simulink model "coba1 - Copy"  (R2021a)
settings: Solver=VariableStepAuto  StartTime=0.0  StopTime=200  RelTol=1e-3
undefined symbols (not defined in the file): Ion, Lithium
libraries: spsSeriesRLCBranchLib x23, spsIdealSwitchLib x14, spsBatteryLib x12, spsDiodeLib x12, spsDCVoltageSourceLib x1, spsGroundLib x1, spsPWMGenerator2LevelLib x1, spspowerguiLib x1
settings Model: Creator=jafar  LastModifiedBy=jafar

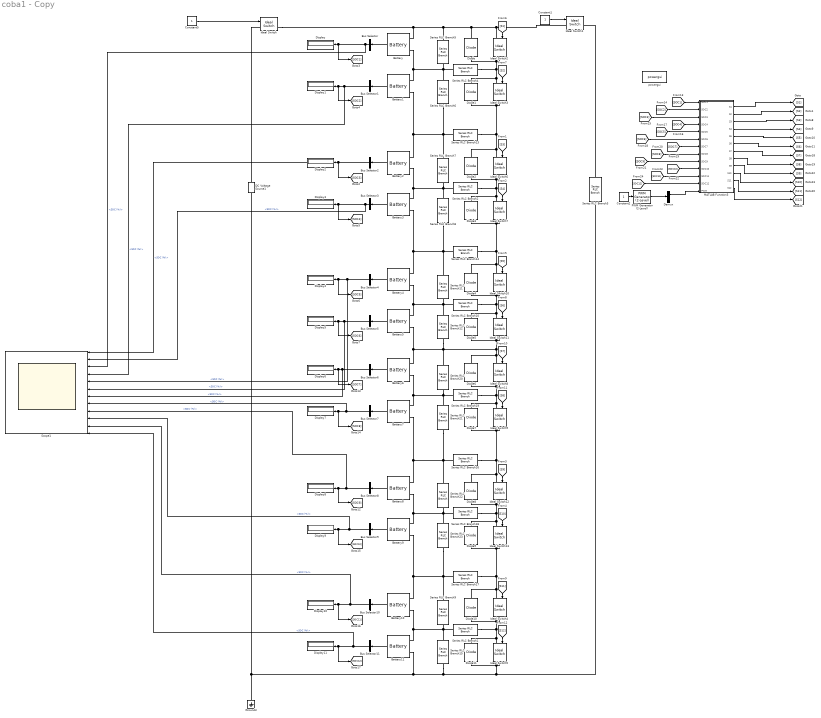
== system coba1 - Copy ==
  Battery : spsBatteryLib/Battery  BatType=Lithium-Ion  ShowTempParam=off  ThermalPreset=no  ShowAgeParam=off  NomV=3.7  NomQ=5.4  SOC=20  Batt_Tr=30  PresetModel=on  MaxQ=5.4  MinV=2.775  FullV=4.3068  Dis_rate=2.3478  R=0.0068519  Normal_OP=4.8835  expZone="[3.9974      0.2653]"  current=[6.5 13 32.5]  Units=Time  Tci=20  NomT=20  T2=-30  MaxQ2=4.8  FullV2=7.1  Normal_OP2=5.655  expZone2="[6.58           1]"  Rca=0.6  ti=2000  Dp=0  Neq0=0  Tsim=1e6  Ta1=25  Qeol=5.4*0.9  Reol=0.013333*1.2  Char_age=[2.3478, 3]  Dis_age=[2.3478, 10]  N1=1500  N2=10500  N3=1000  N4=1400  Ta2=45  N5=950
  Battery1 : spsBatteryLib/Battery  BatType=Lithium-Ion  ShowTempParam=off  ThermalPreset=no  ShowAgeParam=off  NomV=3.7  NomQ=5.4  SOC=30  Batt_Tr=30  PresetModel=on  MaxQ=5.4  MinV=2.775  FullV=4.3068  Dis_rate=2.3478  R=0.0068519  Normal_OP=4.8835  expZone="[3.9974      0.2653]"  current=[6.5 13 32.5]  Units=Time  Tci=20  NomT=20  T2=-30  MaxQ2=4.8  FullV2=7.1  Normal_OP2=5.655  expZone2="[6.58           1]"  Rca=0.6  ti=2000  Dp=0  Neq0=0  Tsim=1e6  Ta1=25  Qeol=5.4*0.9  Reol=0.013333*1.2  Char_age=[2.3478, 3]  Dis_age=[2.3478, 10]  N1=1500  N2=10500  N3=1000  N4=1400  Ta2=45  N5=950
  Battery10 : spsBatteryLib/Battery  BatType=Lithium-Ion  ShowTempParam=off  ThermalPreset=no  ShowAgeParam=off  NomV=3.7  NomQ=5.4  SOC=10  Batt_Tr=30  PresetModel=on  MaxQ=5.4  MinV=2.775  FullV=4.3068  Dis_rate=2.3478  R=0.0068519  Normal_OP=4.8835  expZone="[3.9974      0.2653]"  current=[6.5 13 32.5]  Units=Time  Tci=20  NomT=20  T2=-30  MaxQ2=4.8  FullV2=7.1  Normal_OP2=5.655  expZone2="[6.58           1]"  Rca=0.6  ti=2000  Dp=0  Neq0=0  Tsim=1e6  Ta1=25  Qeol=5.4*0.9  Reol=0.013333*1.2  Char_age=[2.3478, 3]  Dis_age=[2.3478, 10]  N1=1500  N2=10500  N3=1000  N4=1400  Ta2=45  N5=950
  Battery11 : spsBatteryLib/Battery  BatType=Lithium-Ion  ShowTempParam=off  ThermalPreset=no  ShowAgeParam=off  NomV=3.7  NomQ=5.4  SOC=0  Batt_Tr=30  PresetModel=on  MaxQ=5.4  MinV=2.775  FullV=4.3068  Dis_rate=2.3478  R=0.0068519  Normal_OP=4.8835  expZone="[3.9974      0.2653]"  current=[6.5 13 32.5]  Units=Time  Tci=20  NomT=20  T2=-30  MaxQ2=4.8  FullV2=7.1  Normal_OP2=5.655  expZone2="[6.58           1]"  Rca=0.6  ti=2000  Dp=0  Neq0=0  Tsim=1e6  Ta1=25  Qeol=5.4*0.9  Reol=0.013333*1.2  Char_age=[2.3478, 3]  Dis_age=[2.3478, 10]  N1=1500  N2=10500  N3=1000  N4=1400  Ta2=45  N5=950
  Battery2 : spsBatteryLib/Battery  BatType=Lithium-Ion  ShowTempParam=off  ThermalPreset=no  ShowAgeParam=off  NomV=3.7  NomQ=5.4  SOC=40  Batt_Tr=30  PresetModel=on  MaxQ=5.4  MinV=2.775  FullV=4.3068  Dis_rate=2.3478  R=0.0068519  Normal_OP=4.8835  expZone="[3.9974      0.2653]"  current=[6.5 13 32.5]  Units=Time  Tci=20  NomT=20  T2=-30  MaxQ2=4.8  FullV2=7.1  Normal_OP2=5.655  expZone2="[6.58           1]"  Rca=0.6  ti=2000  Dp=0  Neq0=0  Tsim=1e6  Ta1=25  Qeol=5.4*0.9  Reol=0.013333*1.2  Char_age=[2.3478, 3]  Dis_age=[2.3478, 10]  N1=1500  N2=10500  N3=1000  N4=1400  Ta2=45  N5=950
  Battery3 : spsBatteryLib/Battery  BatType=Lithium-Ion  ShowTempParam=off  ThermalPreset=no  ShowAgeParam=off  NomV=3.7  NomQ=5.4  SOC=50  Batt_Tr=30  PresetModel=on  MaxQ=5.4  MinV=2.775  FullV=4.3068  Dis_rate=2.3478  R=0.0068519  Normal_OP=4.8835  expZone="[3.9974      0.2653]"  current=[6.5 13 32.5]  Units=Time  Tci=20  NomT=20  T2=-30  MaxQ2=4.8  FullV2=7.1  Normal_OP2=5.655  expZone2="[6.58           1]"  Rca=0.6  ti=2000  Dp=0  Neq0=0  Tsim=1e6  Ta1=25  Qeol=5.4*0.9  Reol=0.013333*1.2  Char_age=[2.3478, 3]  Dis_age=[2.3478, 10]  N1=1500  N2=10500  N3=1000  N4=1400  Ta2=45  N5=950
  Battery4 : spsBatteryLib/Battery  BatType=Lithium-Ion  ShowTempParam=off  ThermalPreset=no  ShowAgeParam=off  NomV=3.7  NomQ=5.4  SOC=60  Batt_Tr=30  PresetModel=on  MaxQ=5.4  MinV=2.775  FullV=4.3068  Dis_rate=2.3478  R=0.0068519  Normal_OP=4.8835  expZone="[3.9974      0.2653]"  current=[6.5 13 32.5]  Units=Time  Tci=20  NomT=20  T2=-30  MaxQ2=4.8  FullV2=7.1  Normal_OP2=5.655  expZone2="[6.58           1]"  Rca=0.6  ti=2000  Dp=0  Neq0=0  Tsim=1e6  Ta1=25  Qeol=5.4*0.9  Reol=0.013333*1.2  Char_age=[2.3478, 3]  Dis_age=[2.3478, 10]  N1=1500  N2=10500  N3=1000  N4=1400  Ta2=45  N5=950
  Battery5 : spsBatteryLib/Battery  BatType=Lithium-Ion  ShowTempParam=off  ThermalPreset=no  ShowAgeParam=off  NomV=3.7  NomQ=5.4  SOC=70  Batt_Tr=30  PresetModel=on  MaxQ=5.4  MinV=2.775  FullV=4.3068  Dis_rate=2.3478  R=0.0068519  Normal_OP=4.8835  expZone="[3.9974      0.2653]"  current=[6.5 13 32.5]  Units=Time  Tci=20  NomT=20  T2=-30  MaxQ2=4.8  FullV2=7.1  Normal_OP2=5.655  expZone2="[6.58           1]"  Rca=0.6  ti=2000  Dp=0  Neq0=0  Tsim=1e6  Ta1=25  Qeol=5.4*0.9  Reol=0.013333*1.2  Char_age=[2.3478, 3]  Dis_age=[2.3478, 10]  N1=1500  N2=10500  N3=1000  N4=1400  Ta2=45  N5=950
  Battery6 : spsBatteryLib/Battery  BatType=Lithium-Ion  ShowTempParam=off  ThermalPreset=no  ShowAgeParam=off  NomV=3.7  NomQ=5.4  SOC=35  Batt_Tr=30  PresetModel=on  MaxQ=5.4  MinV=2.775  FullV=4.3068  Dis_rate=2.3478  R=0.0068519  Normal_OP=4.8835  expZone="[3.9974      0.2653]"  current=[6.5 13 32.5]  Units=Time  Tci=20  NomT=20  T2=-30  MaxQ2=4.8  FullV2=7.1  Normal_OP2=5.655  expZone2="[6.58           1]"  Rca=0.6  ti=2000  Dp=0  Neq0=0  Tsim=1e6  Ta1=25  Qeol=5.4*0.9  Reol=0.013333*1.2  Char_age=[2.3478, 3]  Dis_age=[2.3478, 10]  N1=1500  N2=10500  N3=1000  N4=1400  Ta2=45  N5=950
  Battery7 : spsBatteryLib/Battery  BatType=Lithium-Ion  ShowTempParam=off  ThermalPreset=no  ShowAgeParam=off  NomV=3.7  NomQ=5.4  SOC=45  Batt_Tr=30  PresetModel=on  MaxQ=5.4  MinV=2.775  FullV=4.3068  Dis_rate=2.3478  R=0.0068519  Normal_OP=4.8835  expZone="[3.9974      0.2653]"  current=[6.5 13 32.5]  Units=Time  Tci=20  NomT=20  T2=-30  MaxQ2=4.8  FullV2=7.1  Normal_OP2=5.655  expZone2="[6.58           1]"  Rca=0.6  ti=2000  Dp=0  Neq0=0  Tsim=1e6  Ta1=25  Qeol=5.4*0.9  Reol=0.013333*1.2  Char_age=[2.3478, 3]  Dis_age=[2.3478, 10]  N1=1500  N2=10500  N3=1000  N4=1400  Ta2=45  N5=950
  Battery8 : spsBatteryLib/Battery  BatType=Lithium-Ion  ShowTempParam=off  ThermalPreset=no  ShowAgeParam=off  NomV=3.7  NomQ=5.4  SOC=30  Batt_Tr=30  PresetModel=on  MaxQ=5.4  MinV=2.775  FullV=4.3068  Dis_rate=2.3478  R=0.0068519  Normal_OP=4.8835  expZone="[3.9974      0.2653]"  current=[6.5 13 32.5]  Units=Time  Tci=20  NomT=20  T2=-30  MaxQ2=4.8  FullV2=7.1  Normal_OP2=5.655  expZone2="[6.58           1]"  Rca=0.6  ti=2000  Dp=0  Neq0=0  Tsim=1e6  Ta1=25  Qeol=5.4*0.9  Reol=0.013333*1.2  Char_age=[2.3478, 3]  Dis_age=[2.3478, 10]  N1=1500  N2=10500  N3=1000  N4=1400  Ta2=45  N5=950
  Battery9 : spsBatteryLib/Battery  BatType=Lithium-Ion  ShowTempParam=off  ThermalPreset=no  ShowAgeParam=off  NomV=3.7  NomQ=5.4  SOC=20  Batt_Tr=30  PresetModel=on  MaxQ=5.4  MinV=2.775  FullV=4.3068  Dis_rate=2.3478  R=0.0068519  Normal_OP=4.8835  expZone="[3.9974      0.2653]"  current=[6.5 13 32.5]  Units=Time  Tci=20  NomT=20  T2=-30  MaxQ2=4.8  FullV2=7.1  Normal_OP2=5.655  expZone2="[6.58           1]"  Rca=0.6  ti=2000  Dp=0  Neq0=0  Tsim=1e6  Ta1=25  Qeol=5.4*0.9  Reol=0.013333*1.2  Char_age=[2.3478, 3]  Dis_age=[2.3478, 10]  N1=1500  N2=10500  N3=1000  N4=1400  Ta2=45  N5=950
  Bus Selector{,1..11} (12 alike) : BusSelector  OutputSignals=SOC (%)
  Constant1 : Constant
  Constant2 : Constant
  Constant5 : Constant
  DC Voltage Source1 : spsDCVoltageSourceLib/DC Voltage Source  Amplitude=72  Measurements=None
  Demux : Demux  Outputs=2
  Diode{,1..11} (12 alike) : spsDiodeLib/Diode  Ron=0.001  Lon=0  Vf=0.8  IC=0  UseSnubber=0  Rs=500  Cs=250e-9  Measurements=off
  Display{,1..11} (12 alike) : Display
  Ground3 : spsGroundLib/Ground  LConnTagsString=a
  Ideal Switch : spsIdealSwitchLib/Ideal Switch  Ron=0.001  Lon=0  IC=0  Rs=1e5  Cs=inf  Measurements=on
  Ideal Switch1 : spsIdealSwitchLib/Ideal Switch  Ron=0.001  Lon=0  IC=0  Rs=1e5  Cs=inf  Measurements=on
  Ideal Switch{2..13} (12 alike) : spsIdealSwitchLib/Ideal Switch  Ron=0.001  Lon=0  IC=0  Rs=1e5  Cs=inf  Measurements=off
  MATLAB Function3 : MATLAB Function  TreatAsAtomicUnit=on
  PWM Generator (2-Level) : spsPWMGenerator2LevelLib/PWM Generator (2-Level)  ModulatorType=Single-phase half-bridge (2 pulses)  ModulatorMode=Unsynchronized  Fc=500  Pc=0  nF=27  MinMax="[ -1  1 ]"  SamplingTechnique=Natural  ModulatingSignals=off  m=0.8  Freq=60  Phase=0  Ts=0  ShowCarrierOutport=off
  Scope1 : Scope  NumInputPorts=12
  Series RLC Branch{1..2,4,10,13..14,16..19} (10 alike) : spsSeriesRLCBranchLib/Series RLC Branch  LConnTagsString=__new0  RConnTagsString=__new0  BranchType=L  Resistance=1  Inductance=1e-3  SetiL0=off  InitialCurrent=0  Capacitance=1e-6  Setx0=off  InitialVoltage=0  Measurements=None
  Series RLC Branch{5..9,11..12,15,20..23} (12 alike) : spsSeriesRLCBranchLib/Series RLC Branch  LConnTagsString=__new0  RConnTagsString=__new0  BranchType=C  Resistance=1  Inductance=1e-3  SetiL0=off  InitialCurrent=0  Capacitance=1e-6  Setx0=off  InitialVoltage=0  Measurements=None
  Series RLC Branch3 : spsSeriesRLCBranchLib/Series RLC Branch  LConnTagsString=__new0  RConnTagsString=__new0  BranchType=R  Resistance=1  Inductance=1e-3  SetiL0=off  InitialCurrent=0  Capacitance=1e-6  Setx0=off  InitialVoltage=0  Measurements=None
  powergui : spspowerguiLib/powergui  Priority=1  SimulationMode=Discrete  SampleTime=50e-5  frequency=60  Iterations=50  frequencyindice=0  Pbase=100e6  ErrMax=1e-4  UnitsV=kV  UnitsW=MW  buscounter=0  FunctionMessages=off  echomessages=off  EnableUseOfTLC=off  CurrentSourceSwitches=off  DisableSnubberDevices=off  DisableRonSwitches=off  DisableVfSwitches=off  DisplayEquations=off  AutomaticDiscreteSolvers=off  SolverType=Tustin/Backward Euler (TBE)  Interpol=off  ExternalGateDelay=off  methode=off  Ts=100  x0status=blocks  SPID=on  SwTol=0  HookPort=off  NonlinearTolerance=1e-4  nMaxIteration=100  ContinueOnMaxIteration=off  RestoreLinks=warning  ResistiveCurrentMeasurement=off  Frange=[0:2:500]  Ylog=off  Xlog=on  ShowGrid=off  save=off  variable=ZData  structure=0  ZoomFFT=off  StartTime=0.0  cycles=1  DisplayStyle=1  fundamental=60  FreqAxis=off  MaxFrequency=1000  frequencyindicesteady=1  RmsSteady=1  display=off
  wires:
  MATLAB Function3/5(S5) -> [S5]
  [S1] -> Ideal Switch2/1
  Bus Selector/1 -> Scope1/3, [SOC1], Display/1  "<SOC (%)>"
  Bus Selector4/1 -> Scope1/5, [SOC5], Display4/1  "<SOC (%)>"
  MATLAB Function3/6(S6) -> [S6]
  Battery2/1 -> Bus Selector2/1
  MATLAB Function3/3(S3) -> [S3]
  [S5] -> Ideal Switch10/1
  MATLAB Function3/4(S4) -> [S4]
  Battery4/1 -> Bus Selector4/1
  Battery5/1 -> Bus Selector5/1
  Bus Selector3/1 -> Scope1/2, [SOC4], Display3/1  "<SOC (%)>"
  Bus Selector5/1 -> Scope1/6, [SOC6], Display5/1  "<SOC (%)>"
  [S4] -> Ideal Switch7/1
  [S6] -> Ideal Switch11/1
  Constant5/1 -> Ideal Switch/1
  Bus Selector1/1 -> Scope1/4, [SOC2], Display1/1  "<SOC (%)>"
  Constant1/1 -> Ideal Switch1/1
  Battery3/1 -> Bus Selector3/1
  [S3] -> Ideal Switch6/1
  Bus Selector2/1 -> Scope1/1, [SOC3], Display2/1  "<SOC (%)>"
  [S2] -> Ideal Switch3/1
  Battery/1 -> Bus Selector/1
  MATLAB Function3/1(S1) -> [S1]
  Battery1/1 -> Bus Selector1/1
  MATLAB Function3/2(S2) -> [S2]
  [SOC1] -> MATLAB Function3/1(SOC1)
  [SOC2] -> MATLAB Function3/2(SOC2)
  [SOC3] -> MATLAB Function3/3(SOC3)
  [SOC4] -> MATLAB Function3/4(SOC4)
  [SOC5] -> MATLAB Function3/5(SOC5)
  [SOC6] -> MATLAB Function3/6(SOC6)
  PWM Generator (2-Level)/1 -> Demux/1
  Constant2/1 -> PWM Generator (2-Level)/1
  Demux/1 -> MATLAB Function3/13(PWM)
  Bus Selector11/1 -> Scope1/12, [SOC12], Display11/1  "<SOC (%)>"
  [S12] -> Ideal Switch5/1
  Bus Selector8/1 -> Scope1/9, [SOC9], Display8/1  "<SOC (%)>"
  Bus Selector6/1 -> Scope1/7, [SOC7], Display6/1  "<SOC (%)>"
  Battery6/1 -> Bus Selector6/1
  [S8] -> Ideal Switch9/1
  Battery7/1 -> Bus Selector7/1
  Battery10/1 -> Bus Selector10/1
  Bus Selector9/1 -> Scope1/10, [SOC10], Display9/1  "<SOC (%)>"
  Bus Selector10/1 -> Scope1/11, [SOC11], Display10/1  "<SOC (%)>"
  [S7] -> Ideal Switch8/1
  Battery8/1 -> Bus Selector8/1
  [S11] -> Ideal Switch4/1
  [S9] -> Ideal Switch12/1
  Bus Selector7/1 -> Scope1/8, [SOC8], Display7/1  "<SOC (%)>"
  Battery11/1 -> Bus Selector11/1
  Battery9/1 -> Bus Selector9/1
  [S10] -> Ideal Switch13/1
  [SOC12] -> MATLAB Function3/12(SOC12)
  [SOC8] -> MATLAB Function3/8(SOC8)
  [SOC11] -> MATLAB Function3/11(SOC11)
  [SOC9] -> MATLAB Function3/9(SOC9)
  [SOC7] -> MATLAB Function3/7(SOC7)
  [SOC10] -> MATLAB Function3/10(SOC10)
  MATLAB Function3/10(S10) -> [S10]
  MATLAB Function3/11(S11) -> [S11]
  MATLAB Function3/9(S9) -> [S9]
  MATLAB Function3/8(S8) -> [S8]
  MATLAB Function3/12(S12) -> [S12]
  MATLAB Function3/7(S7) -> [S7]
  connections:
  Diode1/LConn1 -- Diode2/RConn1 -- Ideal Switch6/LConn1 -- Series RLC Branch13/RConn1 -- Ideal Switch3/RConn1
  Battery5/LConn2 -- Battery6/LConn1 -- Series RLC Branch20/LConn1 -- Series RLC Branch12/RConn1 -- Diode6/RConn1 -- Ideal Switch8/LConn1 -- Ideal Switch11/RConn1 -- Diode5/LConn1
  Series RLC Branch2/LConn1 -- Series RLC Branch8/LConn1 -- Series RLC Branch7/RConn1 -- Battery3/LConn1 -- Battery2/LConn2
  Diode4/LConn1 -- Ideal Switch11/LConn1 -- Diode5/RConn1 -- Series RLC Branch10/RConn1 -- Ideal Switch10/RConn1
  Diode/RConn1 -- Ideal Switch2/LConn1 -- Ideal Switch1/LConn1 -- Battery/LConn1 -- Ideal Switch/RConn1 -- Series RLC Branch5/LConn1
  Series RLC Branch2/RConn1 -- Ideal Switch7/LConn1 -- Diode3/RConn1 -- Ideal Switch6/RConn1 -- Diode2/LConn1
  Series RLC Branch4/LConn1 -- Battery/LConn2 -- Battery1/LConn1 -- Series RLC Branch6/LConn1 -- Series RLC Branch5/RConn1
  Ideal Switch3/LConn1 -- Ideal Switch2/RConn1 -- Diode/LConn1 -- Series RLC Branch4/RConn1 -- Diode1/RConn1
  Series RLC Branch10/LConn1 -- Series RLC Branch12/LConn1 -- Series RLC Branch11/RConn1 -- Battery5/LConn1 -- Battery4/LConn2
  Series RLC Branch3/LConn1 -- Ideal Switch1/RConn1
  Ideal Switch/LConn1 -- DC Voltage Source1/RConn1
  Series RLC Branch7/LConn1 -- Series RLC Branch6/RConn1 -- Battery1/LConn2 -- Battery2/LConn1 -- Series RLC Branch13/LConn1
  Battery3/LConn2 -- Series RLC Branch14/LConn1 -- Series RLC Branch11/LConn1 -- Series RLC Branch8/RConn1 -- Battery4/LConn1
  Ideal Switch7/RConn1 -- Series RLC Branch14/RConn1 -- Diode4/RConn1 -- Ideal Switch10/LConn1 -- Diode3/LConn1
  Series RLC Branch20/RConn1 -- Series RLC Branch19/LConn1 -- Battery6/LConn2 -- Battery7/LConn1 -- Series RLC Branch21/LConn1
  Diode9/LConn1 -- Ideal Switch13/RConn1 -- Series RLC Branch17/RConn1 -- Diode10/RConn1 -- Ideal Switch4/LConn1
  Series RLC Branch16/LConn1 -- Series RLC Branch22/LConn1 -- Series RLC Branch21/RConn1 -- Battery7/LConn2 -- Battery8/LConn1
  Diode11/RConn1 -- Diode10/LConn1 -- Ideal Switch4/RConn1 -- Series RLC Branch1/RConn1 -- Ideal Switch5/LConn1
  Series RLC Branch23/RConn1 -- Battery9/LConn2 -- Battery10/LConn1 -- Series RLC Branch17/LConn1 -- Series RLC Branch9/LConn1
  Battery8/LConn2 -- Series RLC Branch18/LConn1 -- Series RLC Branch23/LConn1 -- Series RLC Branch22/RConn1 -- Battery9/LConn1
  Battery10/LConn2 -- Battery11/LConn1 -- Series RLC Branch1/LConn1 -- Series RLC Branch15/LConn1 -- Series RLC Branch9/RConn1
  Diode9/RConn1 -- Series RLC Branch18/RConn1 -- Ideal Switch12/RConn1 -- Diode8/LConn1 -- Ideal Switch13/LConn1
  Diode7/RConn1 -- Ideal Switch9/LConn1 -- Ideal Switch8/RConn1 -- Diode6/LConn1 -- Series RLC Branch19/RConn1
  Series RLC Branch16/RConn1 -- Diode7/LConn1 -- Ideal Switch9/RConn1 -- Diode8/RConn1 -- Ideal Switch12/LConn1
  Diode11/LConn1 -- Ideal Switch5/RConn1 -- Series RLC Branch3/RConn1 -- Battery11/LConn2 -- DC Voltage Source1/LConn1 -- Ground3/LConn1 -- Series RLC Branch15/RConn1

== matlab function coba1 - Copy/MATLAB Function3 ==
  data: SOC1 input; S1 output; SOC2 input; SOC3 input; SOC4 input; SOC5 input; SOC6 input; SOC7 input; SOC8 input; SOC9 input; SOC10 input; SOC11 input; SOC12 input; S2 output; S3 output; S4 output; S5 output; S6 output; PWM input; S7 output; S8 output; S9 output; S10 output; S11 output; S12 output
function [S1, S2, S3, S4, S5, S6, S7, S8, S9, S10, S11, S12] = fcn(SOC1, SOC2, SOC3, SOC4, SOC5, SOC6, SOC7, SOC8, SOC9, SOC10, SOC11, SOC12, PWM)
    datas = [SOC1, SOC2, SOC3, SOC4, SOC5, SOC6, SOC7, SOC8, SOC9, SOC10, SOC11, SOC12];
    output = zeros(size(datas));
    rata_rata = mean(datas);
    
    for i = 1:length(datas)
        if datas(i) > rata_rata
            output(i) = PWM;
        else
            output(i) = 0;
        end
    end
    
    S1 = output(1);
    S2 = output(2);
    S3 = output(3);
    S4 = output(4);
    S5 = output(5);
    S6 = output(6);
    S7 = output(7);
    S8 = output(8);
    S9 = output(9);
    S10 = output(10);
    S11 = output(11);
    S12 = output(12);
end
